simulink model "Levantamiento_de_cargas_residencial_CR"  (R2018b)
settings: Solver=FixedStepDiscrete  StartTime=0.0  StopTime=1  MaxStep=1e-4  RelTol=1e-3
undefined symbols (not defined in the file): Angle, Magnitude
libraries: powerlib x21
settings Model: Creator=luis  LastModifiedBy=belindabrown
settings OptimizationCC: LifeSpan=inf
settings DebuggingCC: SFExecutionAtInitializationDiag=none
settings SFSimCC: SimUseLocalCustomCode=off
settings RTWCC: RTWUseLocalCustomCode=off
settings CodeAppCC: StateflowObjectComments=on

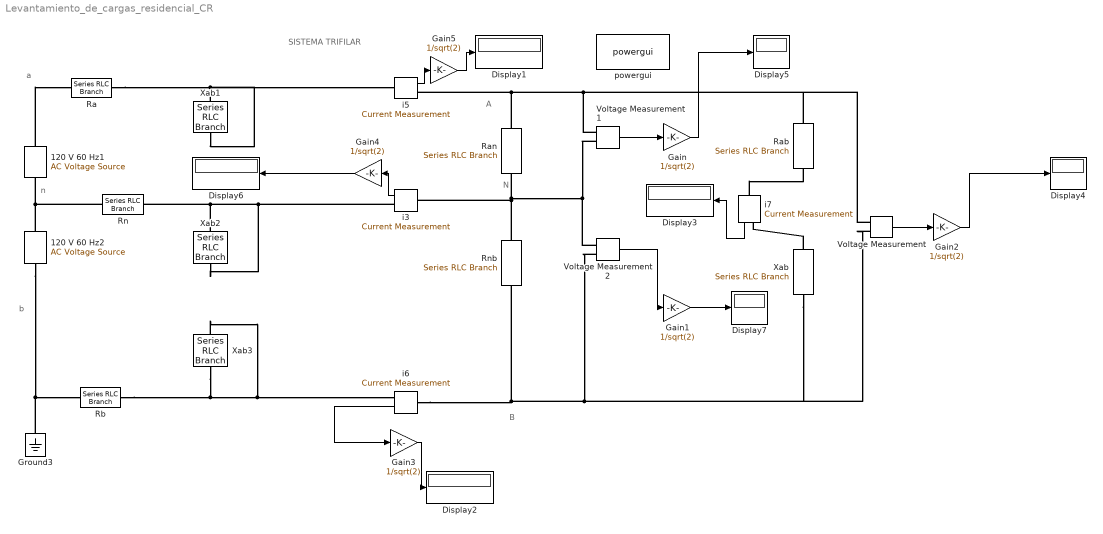
== system Levantamiento_de_cargas_residencial_CR ==
  note: SISTEMA TRIFILAR
  note: B
  note: b
  note: a
  note: n
  note: N
  note: A
  120 V 60 Hz1 : powerlib/Electrical Sources/AC Voltage Source  Description=source block  Amplitude=120*sqrt(2)  Phase=0  Frequency=60  SampleTime=0  Measurements=None  BusType=swing  Pref=10e3  Qref=0  Qmin=-inf  Qmax=+inf
      settings: AttributesFormatString=\n  SourceProductName=Simscape Electrical
  120 V 60 Hz2 : powerlib/Electrical Sources/AC Voltage Source  Description=source block  Amplitude=120*sqrt(2)  Phase=0  Frequency=60  SampleTime=0  Measurements=None  BusType=swing  Pref=10e3  Qref=0  Qmin=-inf  Qmax=+inf
      settings: AttributesFormatString=\n  SourceProductName=Simscape Electrical
  Display{1..7} (7 alike) : Display
  Gain{,1..5} (6 alike) : Gain  Gain=1/sqrt(2)
  Ground3 : powerlib/Elements/Ground  LConnTagsString=a
      settings: SourceProductName=Simscape Electrical
  Ra : powerlib/Elements/Series RLC Branch  LConnTagsString=__new0  RConnTagsString=__new0  BranchType=R  Resistance=0.007  Inductance=[]  SetiL0=off  InitialCurrent=0  Capacitance=[]  Setx0=off  InitialVoltage=0  Measurements=None
      settings: SourceProductName=Simscape Electrical
  Rab : powerlib/Elements/Series RLC Branch  LConnTagsString=__new0  RConnTagsString=__new0  BranchType=R  Resistance=1.74  Inductance=[]  SetiL0=off  InitialCurrent=0  Capacitance=[]  Setx0=off  InitialVoltage=0  Measurements=None
      settings: SourceProductName=Simscape Electrical
  Ran : powerlib/Elements/Series RLC Branch  LConnTagsString=__new0  RConnTagsString=__new0  BranchType=R  Resistance=2.88  Inductance=[]  SetiL0=off  InitialCurrent=0  Capacitance=[]  Setx0=off  InitialVoltage=0  Measurements=None
      settings: SourceProductName=Simscape Electrical
  Rb : powerlib/Elements/Series RLC Branch  LConnTagsString=__new0  RConnTagsString=__new0  BranchType=R  Resistance=0.007  Inductance=[]  SetiL0=off  InitialCurrent=0  Capacitance=[]  Setx0=off  InitialVoltage=0  Measurements=None
      settings: SourceProductName=Simscape Electrical
  Rn : powerlib/Elements/Series RLC Branch  LConnTagsString=__new0  RConnTagsString=__new0  BranchType=R  Resistance=0.017  Inductance=[]  SetiL0=off  InitialCurrent=0  Capacitance=[]  Setx0=off  InitialVoltage=0  Measurements=None
      settings: SourceProductName=Simscape Electrical
  Rnb : powerlib/Elements/Series RLC Branch  LConnTagsString=__new0  RConnTagsString=__new0  BranchType=R  Resistance=1.90  Inductance=[]  SetiL0=off  InitialCurrent=0  Capacitance=[]  Setx0=off  InitialVoltage=0  Measurements=None
      settings: SourceProductName=Simscape Electrical
  Voltage Measurement : powerlib/Measurements/Voltage Measurement  PhasorSimulation=on  OutputType=Magnitude-Angle  PSBequivalent=0
      settings: SourceProductName=Simscape Electrical
  Voltage Measurement1 : powerlib/Measurements/Voltage Measurement  PhasorSimulation=on  OutputType=Magnitude-Angle  PSBequivalent=0
      settings: SourceProductName=Simscape Electrical
  Voltage Measurement2 : powerlib/Measurements/Voltage Measurement  PhasorSimulation=on  OutputType=Magnitude-Angle  PSBequivalent=0
      settings: SourceProductName=Simscape Electrical
  Xab{,1..3} (4 alike) : powerlib/Elements/Series RLC Branch  LConnTagsString=__new0  RConnTagsString=__new0  BranchType=L  Resistance=2  Inductance=0.57/(2*pi*60)  SetiL0=off  InitialCurrent=0  Capacitance=[]  Setx0=off  InitialVoltage=0  Measurements=None
      settings: SourceProductName=Simscape Electrical
  i{3,5..7} (4 alike) : powerlib/Measurements/Current Measurement  Tag=PoWeRsYsTeMmEaSuReMeNt  PhasorSimulation=on  OutputType=Magnitude-Angle  PSBequivalent=0
      settings: SourceProductName=Simscape Electrical
  powergui : powerlib/powergui  Priority=1  SimulationMode=Phasor  SampleTime=50e-6  frequency=60  Iterations=50  frequencyindice=60  Pbase=100e6  ErrMax=1e-4  UnitsV=kV  UnitsW=MW  buscounter=0  FunctionMessages=off  echomessages=off  EnableUseOfTLC=off  CurrentSourceSwitches=off  DisableSnubberDevices=off  DisableRonSwitches=off  DisableVfSwitches=off  DisplayEquations=off  SolverType=Tustin/Backward Euler (TBE)  Interpol=off  ExternalGateDelay=off  methode=off  Ts=100  x0status=blocks  SPID=on  SwTol=0  HookPort=off  RestoreLinks=warning  ResistiveCurrentMeasurement=off  Frange=[0:2:500]  Ylog=off  Xlog=on  ShowGrid=off  save=off  variable=ZData  structure=0  ZoomFFT=off  StartTime=0.0  cycles=1  DisplayStyle=1  fundamental=60  FreqAxis=off  MaxFrequency=1000  frequencyindicesteady=1  RmsSteady=1  display=off
  wires:
  i7/1 -> Display3/1
  Voltage Measurement1/1 -> Gain/1
  Gain/1 -> Display5/1
  Voltage Measurement2/1 -> Gain1/1
  Gain1/1 -> Display7/1
  Voltage Measurement/1 -> Gain2/1
  Gain2/1 -> Display4/1
  Gain5/1 -> Display1/1
  i5/1 -> Gain5/1
  Gain3/1 -> Display2/1
  i6/1 -> Gain3/1
  Gain4/1 -> Display6/1
  i3/1 -> Gain4/1
  connections:
  120 V 60 Hz2/LConn1 -- Ground3/LConn1 -- Rb/LConn1
  120 V 60 Hz2/RConn1 -- Rn/LConn1 -- 120 V 60 Hz1/LConn1
  Rnb/LConn1 -- i3/LConn1 -- Voltage Measurement1/LConn2 -- Voltage Measurement2/LConn1 -- Ran/RConn1
  120 V 60 Hz1/RConn1 -- Ra/LConn1
  Ra/RConn1 -- i5/LConn1 -- Xab1/RConn1 -- Xab1/LConn1
  Ran/LConn1 -- Voltage Measurement1/LConn1 -- Rab/LConn1 -- Voltage Measurement/LConn1 -- i5/RConn1
  i6/LConn1 -- Xab/RConn1 -- Voltage Measurement/LConn2 -- Voltage Measurement2/LConn2 -- Rnb/RConn1
  Rb/RConn1 -- Xab3/RConn1 -- Xab3/LConn1 -- i6/RConn1
  i3/RConn1 -- Xab2/RConn1 -- Rn/RConn1 -- Xab2/LConn1
  i7/LConn1 -- Rab/RConn1
  Xab/LConn1 -- i7/RConn1
